simulink model "MNA1_sim"  (R2014a)
settings: Solver=ode45  StartTime=0.0  StopTime=100  RelTol=1e-3
values from neighbouring files (symbols this model uses):
  MNA1_sys = sys_class    [create_all_sys.m]
settings Model: Creator=UX31  LastModifiedBy=UX31

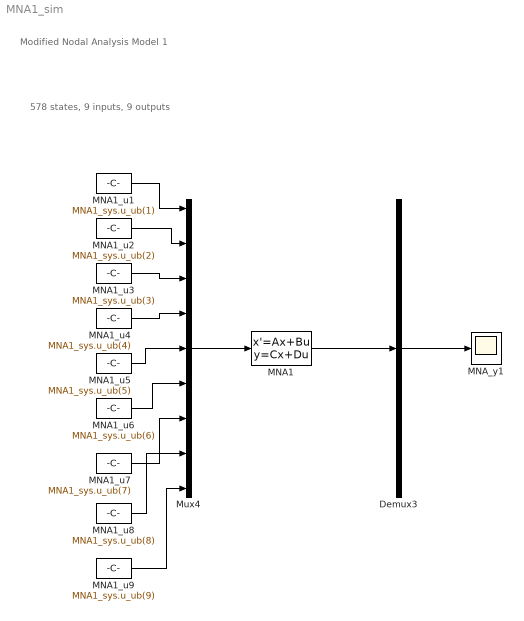
== system MNA1_sim ==
  note: 578 states, 9 inputs, 9 outputs
  note: Modified Nodal Analysis Model 1
  Demux3 : Demux  Outputs=1
  MNA1 : StateSpace  A=MNA1_sys.sys.a  B=MNA1_sys.sys.b  C=MNA1_sys.sys.c  D=MNA1_sys.sys.d  X0=MNA1_sys.x0_lb
  MNA1_u1 : Constant  Value=MNA1_sys.u_ub(1)
  MNA1_u2 : Constant  Value=MNA1_sys.u_ub(2)
  MNA1_u3 : Constant  Value=MNA1_sys.u_ub(3)
  MNA1_u4 : Constant  Value=MNA1_sys.u_ub(4)
  MNA1_u5 : Constant  Value=MNA1_sys.u_ub(5)
  MNA1_u6 : Constant  Value=MNA1_sys.u_ub(6)
  MNA1_u7 : Constant  Value=MNA1_sys.u_ub(7)
  MNA1_u8 : Constant  Value=MNA1_sys.u_ub(8)
  MNA1_u9 : Constant  Value=MNA1_sys.u_ub(9)
  MNA_y1 : Scope
      settings: SaveName=ScopeData13
  Mux4 : Mux  Inputs=9
  wires:
  MNA1_u1/1 -> Mux4/1
  MNA1_u2/1 -> Mux4/2
  MNA1_u3/1 -> Mux4/3
  Mux4/1 -> MNA1/1
  MNA1_u4/1 -> Mux4/4
  MNA1_u5/1 -> Mux4/5
  MNA1_u6/1 -> Mux4/6
  MNA1/1 -> Demux3/1
  Demux3/1 -> MNA_y1/1
  MNA1_u7/1 -> Mux4/7
  MNA1_u8/1 -> Mux4/8
  MNA1_u9/1 -> Mux4/9
